simulink model "graph_import"  (R2019b)
settings: Solver=VariableStepAuto  StartTime=0.0  StopTime=10.0  RelTol=1e-3
undefined symbols (not defined in the file): xc7vx485tffg1157
libraries: ModelComposer x5
settings Model: Creator=abehbood  LastModifiedBy=abehbood

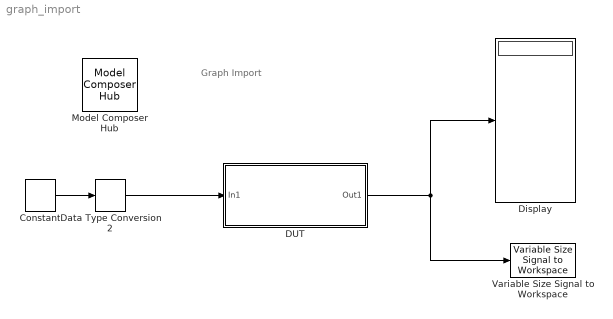
== system graph_import ==
  note: Graph Import
  Constant : ModelComposer/Constant  Value=[1 2 3 4 5 6 7 8 1 2 3 4 5 6 7 8]  SampleTime=1  OutDataType=double  TypeExp=''  Signedness=Signed  WordLength=16  FractionalLength=0  RoundingMode=Truncation to minus infinity  OverflowMode=Wrap around
  DUT : Subsystem
  Data Type Conversion2 : ModelComposer/Data Type Conversion  OutDataType=int16  TypeExp=''  Signedness=Signed  WordLength=16  FractionalLength=0  RoundingMode=Truncation to minus infinity  OverflowMode=Wrap around
  Display : Display
  Model Composer Hub : ModelComposer/Model Composer Hub  CodeGeneration=off  SubsystemName=DUT  TargetDirectory=./code  ExportType=AI Engines  IpVendor=xilinx.com  IpLibrary=hls  IpVersion=1.0  IpHWLanguage=Verilog  AieCompilerOptions={}  CreateTestbench=on  TestbenchStackSize=10  RunAieSim=on  AieSimTimeout=50000  LaunchVitisAnalyzer=off  RunX86Sim=off  X86SimTimeout=10  ProjDevice=xc7vx485tffg1157-1  ProjDevicePart=xc7vx485tffg1157-1  SamplePeriod=-1  ClockFrequency=200  DataPathParallelism=1
  Variable Size Signal to Workspace : ModelComposer/Variable Size Signal to Workspace  VariableNameMask=simout
  wires:
  Constant/1 -> Data Type Conversion2/1
  DUT/1(Out1) -> Display/1, Variable Size Signal to Workspace/1
  Data Type Conversion2/1 -> DUT/1(In1)

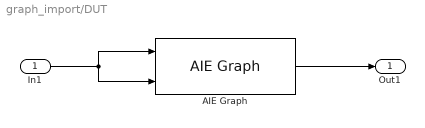
== system graph_import/DUT ==
  In1 : Inport
  AIE Graph : ModelComposer/AIE Graph  PortAttributesTable={ 'Input', 'in1', 'platform.src[0]', 'In1', 'window', 'int16', '16', 'sync', ''; 'Input', 'in2', 'platform.src[1]', 'In2', 'window', 'int16', '16', 'sync', ''; 'Output', 'out1', 'platform.sink[0]', 'Out1', 'window', 'int16', '16', 'sync', '' }  PortAttributesEnablement={'off', 'off', 'off', 'on', 'off', 'off', 'off', 'off', 'off';'off', 'off', 'off', 'on', 'off', 'off', 'off', 'off', 'off';'off', 'off', 'off', 'on', 'off', 'off', 'off', 'off', 'off'}  PortArgDecls={'in window int16 in1'; 'in window int16 in2'; 'out window int16 out1'}  PortNames={'in1'; 'in2'; 'out1'}  PortAliases={'platform.src[0]'; 'platform.src[1]'; 'platform.sink[0]'}  PortGraphPortNames={'In1'; 'In2'; 'Out1'}  PortTypes={'window'; 'window'; 'window'}  PortDataTypes={'int16'; 'int16'; 'int16'}  PortSizes={1.600000000000000000e+01; 1.600000000000000000e+01; 1.600000000000000000e+01}  PortSynchronicities={'sync'; 'sync'; 'sync'}  PortSignalSizes={0.000000000000000000e+00; 0.000000000000000000e+00; 0.000000000000000000e+00}  SimLibPath=''  FunctionTabVisible=on  GraphName=Win_in_win_out  GraphHeaderFiles={'win_in_win_out.h'}  GraphSourceFile=win_in_win_out.cpp  GraphSearchPaths={'./src/kernels/'}  GraphPreProcOptions={}
  Out1 : Outport
  wires:
  In1/1 -> AIE Graph/1, AIE Graph/2
  AIE Graph/1 -> Out1/1
